simulink library "HomeDetector"  (R2018b)
settings: Solver=VariableStepAuto  StartTime=0.0  StopTime=10.0  RelTol=1e-3
settings Model: Creator=nico  LastModifiedBy=Sjoerd

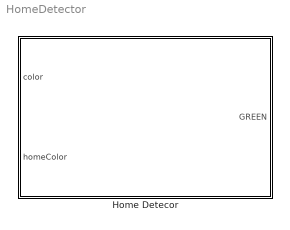
== system HomeDetector ==
  Home Detecor : Stateflow chart  TreatAsAtomicUnit=on

== stateflow chart HomeDetector/Home Detecor ==
  state NotAtHome
    entry:
    GREEN = false
  state PotentialHome
  state Safe
    entry: GREEN = true
    exit: GREEN = false
  (default) -> NotAtHome
  PotentialHome -> NotAtHome [order 1] : [color < homeColor - threshold || color > homeColor + threshold]
  NotAtHome -> PotentialHome : [color >= homeColor - threshold && color <= homeColor + threshold]
  Safe -> PotentialHome : [color < homeColor - threshold || color > homeColor + threshold]
  PotentialHome -> Safe [order 2] : after(delay, msec)
  data: color input; delay constant double =500; threshold constant double =3; GREEN output boolean size=1; homeColor input double =12
